simulink model "model_2_purepursuit"  (R2024b)
settings: Solver=ode23t  StartTime=0.0  StopTime=120  RelTol=1e-3  AbsTol=1e-3  EnableMultiTasking=on
values from neighbouring files (symbols this model uses):
  waypoints = [R*cos(theta)+5, R*sin(theta)]    [init_waypoints.m]
undefined symbols (not defined in the file or in its folder): X, Y, Z
libraries: sm_lib x32, nesl_utility x9, slpidlib x2, robotalgslib x1, sharedtransform x1
(part 2 of 2)

== matlab function model_2_purepursuit/MATLAB Function ==
  data: v input; delta output; w input; L input; v output
function [delta, v] = Diff2Ackermann(v, w, L)
% input: 
%   v - Linear velocity (m/s)
%   w - Angular velocity (rad/s)
%   L -  (m)
%
% output:
%   delta - front whell ratation angel (rad)
%   v     -  velocity(m/s)
if abs(v) < 1e-3
    delta = 0;
else
    delta = atan(L * w / v);   % pure pursuit function
end
